simulink model "carsmodel"  (R2022a)
settings: Solver=VariableStepAuto  StartTime=0  StopTime=100  FixedStep=0.1  MinStep=0.01  RelTol=1e-3  AbsTol=1e-5  EnableMultiTasking=on
undefined symbols (not defined in the file or in its folder): Hecate_brake1, Hecate_brake2, Hecate_freq, Hecate_throttle1, Hecate_throttle2, Hecate_trigger
settings Model: Creator=yoriyuki  LastModifiedBy=fedformi_new
settings SolverCC: AlgebraicLoopSolver=TrustRegion  AutoInsertRateTranBlk=on
settings DataIOCC: ExternalInput=[Throttle, Brake]  FinalStateName=SavePoint  InitialState=SavePoint  SaveOperatingPoint=on  SaveFormat=Array  SignalLogging=off  DSMLogging=off  StateSaveName=x
settings OptimizationCC: LifeSpan=inf
settings DebuggingCC: UnconnectedInputMsg=warning  UnconnectedOutputMsg=warning  UnconnectedLineMsg=warning  AllowSymbolicDim=off  SFUnexpectedBacktrackingDiag=warning  SFNoUnconditionalDefaultTransitionDiag=warning  SFExecutionAtInitializationDiag=none  SFMachineParentedDataDiag=warning  ArithmeticOperatorsInVariantConditions=warning
settings SFSimCC: SimUseLocalCustomCode=off  CustomCodeUndefinedFunction=UseInterfaceOnly
settings RTWCC: RTWUseLocalCustomCode=off  DLArmComputeVersion=19.05
settings CodeAppCC: StateflowObjectComments=on
settings GRTTargetCC: TargetLangStandard=C89/C90 (ANSI)
settings ConfigComp: CovMetricSettings=dw  CovSaveCumulativeToWorkspaceVar=on  CovSaveSingleToWorkspaceVar=on  CovExternalEMLEnable=off

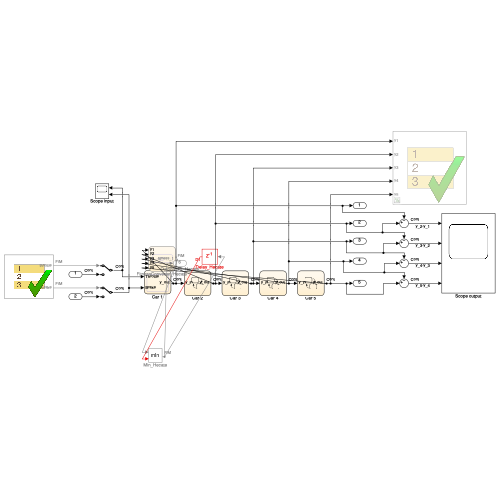
[thumbnail: Simulink's stored preview of the top-level diagram]
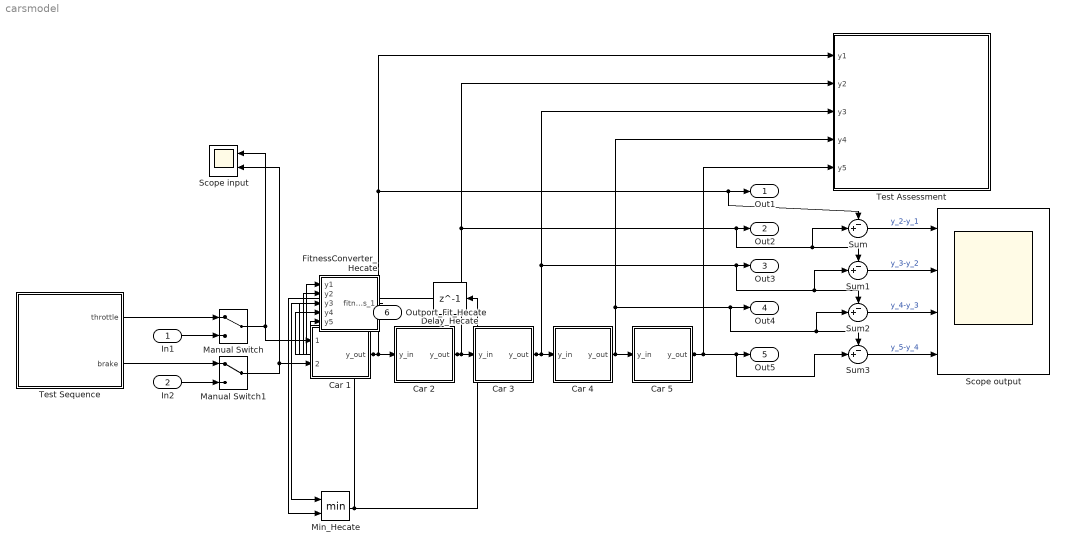
== system carsmodel ==
  In1 : Inport
  In2 : Inport  Port=2
  Car 1 : Stateflow chart  TreatAsAtomicUnit=on
  Car 2 : Stateflow chart  TreatAsAtomicUnit=on
  Car 3 : Stateflow chart  TreatAsAtomicUnit=on
  Car 4 : Stateflow chart  TreatAsAtomicUnit=on
  Car 5 : Stateflow chart  TreatAsAtomicUnit=on
  Delay_Hecate : Delay  DelayLength=1  InitialCondition=Inf
  FitnessConverter_Hecate : Stateflow chart  TreatAsAtomicUnit=on
  Manual Switch : ManualSwitch
  Manual Switch1 : ManualSwitch
  Min_Hecate : MinMax  Inputs=2
  Scope input : Scope  NumInputPorts=2
  Scope output : Scope  NumInputPorts=4
  Sum{,1..3} (4 alike) : Sum  Inputs=-+|
  Test Assessment : Test Sequence  TreatAsAtomicUnit=on
  Test Sequence : Test Sequence  TreatAsAtomicUnit=on
  Out1 : Outport  VectorParamsAs1DForOutWhenUnconnected=off
  Out2 : Outport  Port=2  VectorParamsAs1DForOutWhenUnconnected=off
  Out3 : Outport  Port=3  VectorParamsAs1DForOutWhenUnconnected=off
  Out4 : Outport  Port=4  VectorParamsAs1DForOutWhenUnconnected=off
  Out5 : Outport  Port=5  VectorParamsAs1DForOutWhenUnconnected=off
  Outport_Fit_Hecate : Outport  Port=6
  wires:
  Car 5/1(y_out) -> Test Assessment/5(y5), Sum3/2, Out5/1, FitnessConverter_Hecate/5(y5)
  Car 1/1(y_out) -> Test Assessment/1(y1), Sum/1, Out1/1, Car 2/1(y_in), FitnessConverter_Hecate/1(y1)
  Car 2/1(y_out) -> Test Assessment/2(y2), Sum1/1, Sum/2, Out2/1, Car 3/1(y_in), FitnessConverter_Hecate/2(y2)
  Car 3/1(y_out) -> Test Assessment/3(y3), Sum2/1, Sum1/2, Out3/1, Car 4/1(y_in), FitnessConverter_Hecate/3(y3)
  Car 4/1(y_out) -> Test Assessment/4(y4), Sum3/1, Sum2/2, Out4/1, Car 5/1(y_in), FitnessConverter_Hecate/4(y4)
  Manual Switch/1 -> Scope input/1, Car 1/1(Throttle)
  Manual Switch1/1 -> Car 1/2(Brake), Scope input/2
  In2/1 -> Manual Switch1/2
  In1/1 -> Manual Switch/2
  Test Sequence/1(throttle) -> Manual Switch/1
  Test Sequence/2(brake) -> Manual Switch1/1
  Sum/1 -> Scope output/1  "y_2-y_1"
  Sum1/1 -> Scope output/2  "y_3-y_2"
  Sum2/1 -> Scope output/3  "y_4-y_3"
  Sum3/1 -> Scope output/4  "y_5-y_4"
  FitnessConverter_Hecate/1(fitness_1) -> Min_Hecate/1
  Min_Hecate/1 -> Delay_Hecate/1, Outport_Fit_Hecate/1
  Delay_Hecate/1 -> Min_Hecate/2

== stateflow chart carsmodel/Car 1 ==
  settings: updateMethod=CONTINUOUS
  state Run
    during:
    v_dot = -Throttle - Brake * v;
    y_dot = v;
    y_out = y;
  (default) -> Run
  data: Throttle input; Brake input; y local =0; y_out output; v local =0
  data y settings: updateMethod=SF_CONTINUOUS_TIME_DATA
  data v settings: updateMethod=SF_CONTINUOUS_TIME_DATA

== stateflow chart carsmodel/Car 3 ==
  settings: updateMethod=CONTINUOUS
  state Chasing
    during:
    v_dot = 1;
    y_dot = -v;
    y_out = y;
  state Keeping
    during:
    y_dot = v;
    y_out = y;
  state Braking
    during:
    v_dot = -v;
    y_dot = -v;
    y_out = y;
  (default) -> Keeping
  Chasing -> Keeping : [y - y_in <= 10]
      | % [transition condition]{action}
  Keeping -> Chasing [order 1] : [y - y_in >=15]
  Braking -> Chasing : [y - y_in >= 20]
  Keeping -> Braking [order 2] : [y - y_in <=5]
  data: y_out output; y local double =20; v local =0; y_in input
  data y settings: updateMethod=SF_CONTINUOUS_TIME_DATA
  data v settings: updateMethod=SF_CONTINUOUS_TIME_DATA
  data y_in settings: updateMethod=SF_CONTINUOUS_TIME_DATA

== stateflow chart carsmodel/Car 2 ==
  settings: updateMethod=CONTINUOUS
  state Chasing
    during:
    v_dot = 1;
    y_dot = -v;
    y_out = y;
  state Keeping
    during:
    y_dot = v;
    y_out = y;
  state Braking
    during:
    v_dot = -v;
    y_dot = -v;
    y_out = y;
  (default) -> Keeping
  Chasing -> Keeping : [y - y_in <= 10]
  Keeping -> Chasing [order 1] : [y - y_in >=15]
  Braking -> Chasing : [y - y_in >= 20]
  Keeping -> Braking [order 2] : [y - y_in <=5]
  data: y_out output; y local double =10; v local =0; y_in input
  data y settings: updateMethod=SF_CONTINUOUS_TIME_DATA
  data v settings: updateMethod=SF_CONTINUOUS_TIME_DATA
  data y_in settings: updateMethod=SF_CONTINUOUS_TIME_DATA

== stateflow chart carsmodel/Car 4 ==
  settings: updateMethod=CONTINUOUS
  state Chasing
    during:
    v_dot = 1;
    y_dot = -v;
    y_out = y;
  state Keeping
    during:
    y_dot = v;
    y_out = y;
  state Braking
    during:
    v_dot = -v;
    y_dot = -v;
    y_out = y;
  (default) -> Keeping
  Chasing -> Keeping : [y - y_in <= 10]
      | % [transition condition]{action}
  Keeping -> Chasing [order 1] : [y - y_in >=15]
  Braking -> Chasing : [y - y_in >= 20]
  Keeping -> Braking [order 2] : [y - y_in <=5]
  data: y local double =30; v local =0; y_in input; y_out output
  data y settings: updateMethod=SF_CONTINUOUS_TIME_DATA
  data v settings: updateMethod=SF_CONTINUOUS_TIME_DATA
  data y_in settings: updateMethod=SF_CONTINUOUS_TIME_DATA

== stateflow chart carsmodel/Car 5 ==
  settings: updateMethod=CONTINUOUS
  state Keeping
    during:
    y_dot = v;
    y_out = y;
  state Chasing
    during:
    v_dot = 1;
    y_dot = -v;
    y_out = y;
  state Braking
    during:
    v_dot = -v;
    y_dot = -v;
    y_out = y;
  (default) -> Keeping
  Chasing -> Keeping : [y - y_in <= 10]
      | % [transition condition]{action}
  Keeping -> Chasing [order 1] : [y - y_in >=15]
  Braking -> Chasing : [y - y_in >= 20]
  Keeping -> Braking [order 2] : [y - y_in <=5]
  data: y_out output; y local double =40; v local =0; y_in input
  data y settings: updateMethod=SF_CONTINUOUS_TIME_DATA
  data v settings: updateMethod=SF_CONTINUOUS_TIME_DATA
  data y_in settings: updateMethod=SF_CONTINUOUS_TIME_DATA

== stateflow chart carsmodel/Test Assessment ==
  state CC1
    state step_1
      state step_1_1
        verify(y5-y4<=40)
      state step_1_2
      (default) -> (junction 55)
      CC1.step_1 -> (junction 55)
      (junction 55) -> (junction 56) [order 1] : [t >= 0 && t <=100
          | ]
      (junction 56) -> CC1.step_1.step_1_1 [order 1] : [~in(CC1.step_1.step_1_1)]
      (junction 56) -> (junction 59) [order 2]
      (junction 64) -> (junction 65)
      (junction 65) -> CC1.step_1.step_1_2 [order 1] : [~in(CC1.step_1.step_1_2)]
      (junction 65) -> (junction 68) [order 2]
      (junction 55) -> (junction 64) [order 2]
    (default) -> CC1.step_1
  state CCX
    state step_1
      state step_1_1
        verify(y2-y1>7.5 && y3-y2>7.5 && y4-y3>7.5 && y5-y4>7.5)
      state step_1_2
      CCX.step_1 -> (junction 162)
      (default) -> (junction 162)
      (junction 162) -> (junction 163) [order 1] : [t>=0 && t<=50
          | ]
      (junction 163) -> CCX.step_1.step_1_1 [order 1] : [~in(CCX.step_1.step_1_1)]
      (junction 163) -> (junction 166) [order 2]
      (junction 210) -> (junction 211)
      (junction 211) -> CCX.step_1.step_1_2 [order 1] : [~in(CCX.step_1.step_1_2)]
      (junction 211) -> (junction 214) [order 2]
      (junction 162) -> (junction 210) [order 2]
    (default) -> CCX.step_1
  (default) -> CC1 [order 1] : [Active_Scenario_Index == 1]
  (default) -> CCX [order 2] : {assert(Active_Scenario_Index == 2,'The value of Scenario Parameter ''Active_Scenario_Index'' is not valid. Use the index of the scenario to specify it.')}
  data: y1 input; y2 input; y3 input; y4 input; y5 input; Active_Scenario_Index parameter =1

== stateflow chart carsmodel/Test Sequence ==
  state step_1
    throttle = Hecate_throttle1;
    brake  = Hecate_brake1;
  state step_2
    throttle = 0.5+Hecate_throttle2*sin(2*pi*Hecate_freq*t);
    throttle = 0.5+Hecate_brake2*cos(2*pi*Hecate_freq*t);
  (default) -> step_1
  step_1 -> step_2 : [
      | t > Hecate_trigger
      | ]
  data: throttle output; brake output; Hecate_throttle1 parameter; Hecate_trigger parameter; Hecate_brake1 parameter; Hecate_throttle2 parameter; Hecate_brake2 parameter; Hecate_freq parameter

== stateflow chart carsmodel/FitnessConverter_Hecate ==
  state step_1
    fitness_1 = Inf;
    state step_1_1
      fitness_1 = 40-(y5-y4);
    state step_1_2
      fitness_1 = Inf;
    (default) -> (junction 4)
    step_1_2 -> (junction 4) : [(t >= 0 && t <=100)]
    (junction 4) -> step_1_1 [order 1] : [t >= 0 && t <=100]
    (junction 4) -> step_1_2 [order 2] : []
    step_1_1 -> (junction 4) : [~(t >= 0 && t <=100)]
  (default) -> step_1
  data: y1 input; y2 input; y3 input; y4 input; y5 input; fitness_1 output
